simulink model "Supported_and_unsupported_combinations"  (Simulink 7.8)
settings: Solver=ode15s  StartTime=0.0  StopTime=inf  MaxStep=0.2  RelTol=1e-3
undefined symbols (not defined in the file): Engine, Engine1, Engine2, Engine3, Engine4, Engine5, Engine6, Engine7, Engine8, Engine9
libraries: sFunctionBlocks x32
(part 2 of 4)

== system Supported_and_unsupported_combinations/BoundaryConditionsConstant ==
  inflow : Inport
  Constant : Constant  Value=0
  Constant1 : Constant  Value=Pbc
  Constant2 : Constant  Value=Tbc
  Constant3 : Constant  Value=XO2bc
  Conversion_XO2_lambda : Fcn  Expr=u(1) / 0.231362 * (1 + 14.59) / (14.59 * (1 - u(1) / 0.231362))+1
  Ground : Ground
  Saturation : Saturate  UpperLimit=0.2313  LowerLimit=0
  Terminator : Terminator
  outflow : Outport
  tag scope: none=global
  wires:
  Constant1/1 -> [none]
  Constant2/1 -> [none]
  Constant3/1 -> [none], Saturation/1
  inflow/1 -> Terminator/1
  Ground/1 -> outflow/1
  Conversion_XO2_lambda/1 -> [none]
  Constant/1 -> [none]
  Saturation/1 -> Conversion_XO2_lambda/1

== system Supported_and_unsupported_combinations/BoundaryConditionsConstant1 ==
  inflow : Inport
  Constant : Constant  Value=0
  Constant1 : Constant  Value=Pbc
  Constant2 : Constant  Value=Tbc
  Constant3 : Constant  Value=XO2bc
  Conversion_XO2_lambda : Fcn  Expr=u(1) / 0.231362 * (1 + 14.59) / (14.59 * (1 - u(1) / 0.231362))+1
  Ground : Ground
  Saturation : Saturate  UpperLimit=0.2313  LowerLimit=0
  Terminator : Terminator
  outflow : Outport
  tag scope: none=global
  wires:
  Saturation/1 -> Conversion_XO2_lambda/1
  Constant/1 -> [none]
  Conversion_XO2_lambda/1 -> [none]
  Ground/1 -> outflow/1
  inflow/1 -> Terminator/1
  Constant3/1 -> Saturation/1, [none]
  Constant2/1 -> [none]
  Constant1/1 -> [none]

== system Supported_and_unsupported_combinations/BoundaryConditionsConstant2 ==
  inflow : Inport
  Constant : Constant  Value=0
  Constant1 : Constant  Value=Pbc
  Constant2 : Constant  Value=Tbc
  Constant3 : Constant  Value=XO2bc
  Conversion_XO2_lambda : Fcn  Expr=u(1) / 0.231362 * (1 + 14.59) / (14.59 * (1 - u(1) / 0.231362))+1
  Ground : Ground
  Saturation : Saturate  UpperLimit=0.2313  LowerLimit=0
  Terminator : Terminator
  outflow : Outport
  tag scope: none=global
  wires:
  Constant1/1 -> [none]
  Constant2/1 -> [none]
  Constant3/1 -> [none], Saturation/1
  inflow/1 -> Terminator/1
  Ground/1 -> outflow/1
  Conversion_XO2_lambda/1 -> [none]
  Constant/1 -> [none]
  Saturation/1 -> Conversion_XO2_lambda/1

== system Supported_and_unsupported_combinations/BoundaryConditionsConstant3 ==
  inflow : Inport
  Constant : Constant  Value=0
  Constant1 : Constant  Value=Pbc
  Constant2 : Constant  Value=Tbc
  Constant3 : Constant  Value=XO2bc
  Conversion_XO2_lambda : Fcn  Expr=u(1) / 0.231362 * (1 + 14.59) / (14.59 * (1 - u(1) / 0.231362))+1
  Ground : Ground
  Saturation : Saturate  UpperLimit=0.2313  LowerLimit=0
  Terminator : Terminator
  outflow : Outport
  tag scope: none=global
  wires:
  Saturation/1 -> Conversion_XO2_lambda/1
  Constant/1 -> [none]
  Conversion_XO2_lambda/1 -> [none]
  Ground/1 -> outflow/1
  inflow/1 -> Terminator/1
  Constant3/1 -> Saturation/1, [none]
  Constant2/1 -> [none]
  Constant1/1 -> [none]

== system Supported_and_unsupported_combinations/BoundaryConditionsConstant4 ==
  inflow : Inport
  Constant : Constant  Value=0
  Constant1 : Constant  Value=Pbc
  Constant2 : Constant  Value=Tbc
  Constant3 : Constant  Value=XO2bc
  Conversion_XO2_lambda : Fcn  Expr=u(1) / 0.231362 * (1 + 14.59) / (14.59 * (1 - u(1) / 0.231362))+1
  Ground : Ground
  Saturation : Saturate  UpperLimit=0.2313  LowerLimit=0
  Terminator : Terminator
  outflow : Outport
  tag scope: none=global
  wires:
  Constant1/1 -> [none]
  Constant2/1 -> [none]
  Constant3/1 -> [none], Saturation/1
  inflow/1 -> Terminator/1
  Ground/1 -> outflow/1
  Conversion_XO2_lambda/1 -> [none]
  Constant/1 -> [none]
  Saturation/1 -> Conversion_XO2_lambda/1

== system Supported_and_unsupported_combinations/BoundaryConditionsConstant5 ==
  inflow : Inport
  Constant : Constant  Value=0
  Constant1 : Constant  Value=Pbc
  Constant2 : Constant  Value=Tbc
  Constant3 : Constant  Value=XO2bc
  Conversion_XO2_lambda : Fcn  Expr=u(1) / 0.231362 * (1 + 14.59) / (14.59 * (1 - u(1) / 0.231362))+1
  Ground : Ground
  Saturation : Saturate  UpperLimit=0.2313  LowerLimit=0
  Terminator : Terminator
  outflow : Outport
  tag scope: none=global
  wires:
  Saturation/1 -> Conversion_XO2_lambda/1
  Constant/1 -> [none]
  Conversion_XO2_lambda/1 -> [none]
  Ground/1 -> outflow/1
  inflow/1 -> Terminator/1
  Constant3/1 -> Saturation/1, [none]
  Constant2/1 -> [none]
  Constant1/1 -> [none]

== system Supported_and_unsupported_combinations/BoundaryConditionsConstant6 ==
  inflow : Inport
  Constant : Constant  Value=0
  Constant1 : Constant  Value=Pbc
  Constant2 : Constant  Value=Tbc
  Constant3 : Constant  Value=XO2bc
  Conversion_XO2_lambda : Fcn  Expr=u(1) / 0.231362 * (1 + 14.59) / (14.59 * (1 - u(1) / 0.231362))+1
  Ground : Ground
  Saturation : Saturate  UpperLimit=0.2313  LowerLimit=0
  Terminator : Terminator
  outflow : Outport
  tag scope: none=global
  wires:
  Saturation/1 -> Conversion_XO2_lambda/1
  Constant/1 -> [none]
  Conversion_XO2_lambda/1 -> [none]
  Ground/1 -> outflow/1
  inflow/1 -> Terminator/1
  Constant3/1 -> Saturation/1, [none]
  Constant2/1 -> [none]
  Constant1/1 -> [none]

== system Supported_and_unsupported_combinations/BoundaryConditionsConstant7 ==
  inflow : Inport
  Constant : Constant  Value=0
  Constant1 : Constant  Value=Pbc
  Constant2 : Constant  Value=Tbc
  Constant3 : Constant  Value=XO2bc
  Conversion_XO2_lambda : Fcn  Expr=u(1) / 0.231362 * (1 + 14.59) / (14.59 * (1 - u(1) / 0.231362))+1
  Ground : Ground
  Saturation : Saturate  UpperLimit=0.2313  LowerLimit=0
  Terminator : Terminator
  outflow : Outport
  tag scope: none=global
  wires:
  Saturation/1 -> Conversion_XO2_lambda/1
  Constant/1 -> [none]
  Conversion_XO2_lambda/1 -> [none]
  Ground/1 -> outflow/1
  inflow/1 -> Terminator/1
  Constant3/1 -> Saturation/1, [none]
  Constant2/1 -> [none]
  Constant1/1 -> [none]

== system Supported_and_unsupported_combinations/BoundaryConditionsConstant8 ==
  inflow : Inport
  Constant : Constant  Value=0
  Constant1 : Constant  Value=Pbc
  Constant2 : Constant  Value=Tbc
  Constant3 : Constant  Value=XO2bc
  Conversion_XO2_lambda : Fcn  Expr=u(1) / 0.231362 * (1 + 14.59) / (14.59 * (1 - u(1) / 0.231362))+1
  Ground : Ground
  Saturation : Saturate  UpperLimit=0.2313  LowerLimit=0
  Terminator : Terminator
  outflow : Outport
  tag scope: none=global
  wires:
  Constant1/1 -> [none]
  Constant2/1 -> [none]
  Constant3/1 -> [none], Saturation/1
  inflow/1 -> Terminator/1
  Ground/1 -> outflow/1
  Conversion_XO2_lambda/1 -> [none]
  Constant/1 -> [none]
  Saturation/1 -> Conversion_XO2_lambda/1

== system Supported_and_unsupported_combinations/BoundaryConditionsConstant9 ==
  inflow : Inport
  Constant : Constant  Value=0
  Constant1 : Constant  Value=Pbc
  Constant2 : Constant  Value=Tbc
  Constant3 : Constant  Value=XO2bc
  Conversion_XO2_lambda : Fcn  Expr=u(1) / 0.231362 * (1 + 14.59) / (14.59 * (1 - u(1) / 0.231362))+1
  Ground : Ground
  Saturation : Saturate  UpperLimit=0.2313  LowerLimit=0
  Terminator : Terminator
  outflow : Outport
  tag scope: none=global
  wires:
  Constant1/1 -> [none]
  Constant2/1 -> [none]
  Constant3/1 -> [none], Saturation/1
  inflow/1 -> Terminator/1
  Ground/1 -> outflow/1
  Conversion_XO2_lambda/1 -> [none]
  Constant/1 -> [none]
  Saturation/1 -> Conversion_XO2_lambda/1

== system Supported_and_unsupported_combinations/Engine ==
  inflow : Inport
  OmegaEng : Inport  Port=2
  IQ : Inport  Port=3
  uSOI : Inport  Port=4
  uPR : Inport  Port=5
  Constant : Constant  Value=0
  Constant1 : Constant  Value=0
  Engine : Subsystem
  ExhaustManifold : Subsystem
  IntakeManifold : Subsystem
  outflow : Outport
  tag scope: Engine_EngineSpeed=global, Engine_FuelMassflow=global
  wires:
  uPR/1 -> Engine/10(uPR)
  Constant/1 -> Engine/9(uECA)
  Constant1/1 -> Engine/8(uICA)
  Engine/5(Mfuel) -> ExhaustManifold/5(Mfuel), [Engine_FuelMassflow]
  Engine/4(outflow) -> ExhaustManifold/4(inflow)
  IntakeManifold/3(outflow) -> Engine/4(inflow)
  IntakeManifold/1(Pim) -> Engine/1(Pin)
  ExhaustManifold/1(Pout) -> Engine/2(Pout)
  Engine/3(XO2out) -> ExhaustManifold/3(XO2in)
  IntakeManifold/2(XO2out) -> Engine/3(XO2in)
  Engine/2(Tout) -> ExhaustManifold/2(Tin)
  Engine/1(Meng) -> IntakeManifold/1(Mout), ExhaustManifold/1(Meng)
  ExhaustManifold/2(outflow) -> outflow/1
  inflow/1 -> IntakeManifold/2(inflow)
  OmegaEng/1 -> Engine/5(OmegaEng), [Engine_EngineSpeed]
  uSOI/1 -> Engine/7(uSOI)
  IQ/1 -> Engine/6(IQ)

== system Supported_and_unsupported_combinations/Engine1 ==
  inflow : Inport
  OmegaEng : Inport  Port=2
  IQ : Inport  Port=3
  uSOI : Inport  Port=4
  uPR : Inport  Port=5
  Constant : Constant  Value=0
  Constant1 : Constant  Value=0
  Engine : Subsystem
  ExhaustManifold : Subsystem
  IntakeManifold : Subsystem
  outflow : Outport
  tag scope: Engine_EngineSpeed=global, Engine_FuelMassflow=global
  wires:
  IQ/1 -> Engine/6(IQ)
  uSOI/1 -> Engine/7(uSOI)
  OmegaEng/1 -> [Engine_EngineSpeed], Engine/5(OmegaEng)
  inflow/1 -> IntakeManifold/2(inflow)
  ExhaustManifold/2(outflow) -> outflow/1
  Engine/1(Meng) -> ExhaustManifold/1(Meng), IntakeManifold/1(Mout)
  Engine/2(Tout) -> ExhaustManifold/2(Tin)
  IntakeManifold/2(XO2out) -> Engine/3(XO2in)
  Engine/3(XO2out) -> ExhaustManifold/3(XO2in)
  ExhaustManifold/1(Pout) -> Engine/2(Pout)
  IntakeManifold/1(Pim) -> Engine/1(Pin)
  IntakeManifold/3(outflow) -> Engine/4(inflow)
  Engine/4(outflow) -> ExhaustManifold/4(inflow)
  Engine/5(Mfuel) -> [Engine_FuelMassflow], ExhaustManifold/5(Mfuel)
  Constant1/1 -> Engine/8(uICA)
  Constant/1 -> Engine/9(uECA)
  uPR/1 -> Engine/10(uPR)

== system Supported_and_unsupported_combinations/Engine2 ==
  inflow : Inport
  OmegaEng : Inport  Port=2
  IQ : Inport  Port=3
  uSOI : Inport  Port=4
  uPR : Inport  Port=5
  Constant : Constant  Value=0
  Constant1 : Constant  Value=0
  Engine : Subsystem
  ExhaustManifold : Subsystem
  IntakeManifold : Subsystem
  outflow : Outport
  tag scope: Engine_EngineSpeed=global, Engine_FuelMassflow=global
  wires:
  IQ/1 -> Engine/6(IQ)
  uSOI/1 -> Engine/7(uSOI)
  OmegaEng/1 -> [Engine_EngineSpeed], Engine/5(OmegaEng)
  inflow/1 -> IntakeManifold/2(inflow)
  ExhaustManifold/2(outflow) -> outflow/1
  Engine/1(Meng) -> ExhaustManifold/1(Meng), IntakeManifold/1(Mout)
  Engine/2(Tout) -> ExhaustManifold/2(Tin)
  IntakeManifold/2(XO2out) -> Engine/3(XO2in)
  Engine/3(XO2out) -> ExhaustManifold/3(XO2in)
  ExhaustManifold/1(Pout) -> Engine/2(Pout)
  IntakeManifold/1(Pim) -> Engine/1(Pin)
  IntakeManifold/3(outflow) -> Engine/4(inflow)
  Engine/4(outflow) -> ExhaustManifold/4(inflow)
  Engine/5(Mfuel) -> [Engine_FuelMassflow], ExhaustManifold/5(Mfuel)
  Constant1/1 -> Engine/8(uICA)
  Constant/1 -> Engine/9(uECA)
  uPR/1 -> Engine/10(uPR)

== system Supported_and_unsupported_combinations/Engine3 ==
  inflow : Inport
  OmegaEng : Inport  Port=2
  IQ : Inport  Port=3
  uSOI : Inport  Port=4
  uPR : Inport  Port=5
  Constant : Constant  Value=0
  Constant1 : Constant  Value=0
  Engine : Subsystem
  ExhaustManifold : Subsystem
  IntakeManifold : Subsystem
  outflow : Outport
  tag scope: Engine_EngineSpeed=global, Engine_FuelMassflow=global
  wires:
  uPR/1 -> Engine/10(uPR)
  Constant/1 -> Engine/9(uECA)
  Constant1/1 -> Engine/8(uICA)
  Engine/5(Mfuel) -> ExhaustManifold/5(Mfuel), [Engine_FuelMassflow]
  Engine/4(outflow) -> ExhaustManifold/4(inflow)
  IntakeManifold/3(outflow) -> Engine/4(inflow)
  IntakeManifold/1(Pim) -> Engine/1(Pin)
  ExhaustManifold/1(Pout) -> Engine/2(Pout)
  Engine/3(XO2out) -> ExhaustManifold/3(XO2in)
  IntakeManifold/2(XO2out) -> Engine/3(XO2in)
  Engine/2(Tout) -> ExhaustManifold/2(Tin)
  Engine/1(Meng) -> IntakeManifold/1(Mout), ExhaustManifold/1(Meng)
  ExhaustManifold/2(outflow) -> outflow/1
  inflow/1 -> IntakeManifold/2(inflow)
  OmegaEng/1 -> Engine/5(OmegaEng), [Engine_EngineSpeed]
  uSOI/1 -> Engine/7(uSOI)
  IQ/1 -> Engine/6(IQ)

== system Supported_and_unsupported_combinations/Engine4 ==
  inflow : Inport
  OmegaEng : Inport  Port=2
  IQ : Inport  Port=3
  uSOI : Inport  Port=4
  uPR : Inport  Port=5
  Constant : Constant  Value=0
  Constant1 : Constant  Value=0
  Engine : Subsystem
  ExhaustManifold : Subsystem
  IntakeManifold : Subsystem
  outflow : Outport
  tag scope: Engine_EngineSpeed=global, Engine_FuelMassflow=global
  wires:
  IQ/1 -> Engine/6(IQ)
  uSOI/1 -> Engine/7(uSOI)
  OmegaEng/1 -> [Engine_EngineSpeed], Engine/5(OmegaEng)
  inflow/1 -> IntakeManifold/2(inflow)
  ExhaustManifold/2(outflow) -> outflow/1
  Engine/1(Meng) -> ExhaustManifold/1(Meng), IntakeManifold/1(Mout)
  Engine/2(Tout) -> ExhaustManifold/2(Tin)
  IntakeManifold/2(XO2out) -> Engine/3(XO2in)
  Engine/3(XO2out) -> ExhaustManifold/3(XO2in)
  ExhaustManifold/1(Pout) -> Engine/2(Pout)
  IntakeManifold/1(Pim) -> Engine/1(Pin)
  IntakeManifold/3(outflow) -> Engine/4(inflow)
  Engine/4(outflow) -> ExhaustManifold/4(inflow)
  Engine/5(Mfuel) -> [Engine_FuelMassflow], ExhaustManifold/5(Mfuel)
  Constant1/1 -> Engine/8(uICA)
  Constant/1 -> Engine/9(uECA)
  uPR/1 -> Engine/10(uPR)

== system Supported_and_unsupported_combinations/Engine5 ==
  inflow : Inport
  OmegaEng : Inport  Port=2
  IQ : Inport  Port=3
  uSOI : Inport  Port=4
  uPR : Inport  Port=5
  Constant : Constant  Value=0
  Constant1 : Constant  Value=0
  Engine : Subsystem
  ExhaustManifold : Subsystem
  IntakeManifold : Subsystem
  outflow : Outport
  tag scope: Engine_EngineSpeed=global, Engine_FuelMassflow=global
  wires:
  uPR/1 -> Engine/10(uPR)
  Constant/1 -> Engine/9(uECA)
  Constant1/1 -> Engine/8(uICA)
  Engine/5(Mfuel) -> ExhaustManifold/5(Mfuel), [Engine_FuelMassflow]
  Engine/4(outflow) -> ExhaustManifold/4(inflow)
  IntakeManifold/3(outflow) -> Engine/4(inflow)
  IntakeManifold/1(Pim) -> Engine/1(Pin)
  ExhaustManifold/1(Pout) -> Engine/2(Pout)
  Engine/3(XO2out) -> ExhaustManifold/3(XO2in)
  IntakeManifold/2(XO2out) -> Engine/3(XO2in)
  Engine/2(Tout) -> ExhaustManifold/2(Tin)
  Engine/1(Meng) -> IntakeManifold/1(Mout), ExhaustManifold/1(Meng)
  ExhaustManifold/2(outflow) -> outflow/1
  inflow/1 -> IntakeManifold/2(inflow)
  OmegaEng/1 -> Engine/5(OmegaEng), [Engine_EngineSpeed]
  uSOI/1 -> Engine/7(uSOI)
  IQ/1 -> Engine/6(IQ)

== system Supported_and_unsupported_combinations/Engine6 ==
  inflow : Inport
  OmegaEng : Inport  Port=2
  IQ : Inport  Port=3
  uSOI : Inport  Port=4
  uPR : Inport  Port=5
  Constant : Constant  Value=0
  Constant1 : Constant  Value=0
  Engine : Subsystem
  ExhaustManifold : Subsystem
  IntakeManifold : Subsystem
  outflow : Outport
  tag scope: Engine_EngineSpeed=global, Engine_FuelMassflow=global
  wires:
  uPR/1 -> Engine/10(uPR)
  Constant/1 -> Engine/9(uECA)
  Constant1/1 -> Engine/8(uICA)
  Engine/5(Mfuel) -> ExhaustManifold/5(Mfuel), [Engine_FuelMassflow]
  Engine/4(outflow) -> ExhaustManifold/4(inflow)
  IntakeManifold/3(outflow) -> Engine/4(inflow)
  IntakeManifold/1(Pim) -> Engine/1(Pin)
  ExhaustManifold/1(Pout) -> Engine/2(Pout)
  Engine/3(XO2out) -> ExhaustManifold/3(XO2in)
  IntakeManifold/2(XO2out) -> Engine/3(XO2in)
  Engine/2(Tout) -> ExhaustManifold/2(Tin)
  Engine/1(Meng) -> IntakeManifold/1(Mout), ExhaustManifold/1(Meng)
  ExhaustManifold/2(outflow) -> outflow/1
  inflow/1 -> IntakeManifold/2(inflow)
  OmegaEng/1 -> Engine/5(OmegaEng), [Engine_EngineSpeed]
  uSOI/1 -> Engine/7(uSOI)
  IQ/1 -> Engine/6(IQ)

== system Supported_and_unsupported_combinations/Engine7 ==
  inflow : Inport
  OmegaEng : Inport  Port=2
  IQ : Inport  Port=3
  uSOI : Inport  Port=4
  uPR : Inport  Port=5
  Constant : Constant  Value=0
  Constant1 : Constant  Value=0
  Engine : Subsystem
  ExhaustManifold : Subsystem
  IntakeManifold : Subsystem
  outflow : Outport
  tag scope: Engine_EngineSpeed=global, Engine_FuelMassflow=global
  wires:
  IQ/1 -> Engine/6(IQ)
  uSOI/1 -> Engine/7(uSOI)
  OmegaEng/1 -> [Engine_EngineSpeed], Engine/5(OmegaEng)
  inflow/1 -> IntakeManifold/2(inflow)
  ExhaustManifold/2(outflow) -> outflow/1
  Engine/1(Meng) -> ExhaustManifold/1(Meng), IntakeManifold/1(Mout)
  Engine/2(Tout) -> ExhaustManifold/2(Tin)
  IntakeManifold/2(XO2out) -> Engine/3(XO2in)
  Engine/3(XO2out) -> ExhaustManifold/3(XO2in)
  ExhaustManifold/1(Pout) -> Engine/2(Pout)
  IntakeManifold/1(Pim) -> Engine/1(Pin)
  IntakeManifold/3(outflow) -> Engine/4(inflow)
  Engine/4(outflow) -> ExhaustManifold/4(inflow)
  Engine/5(Mfuel) -> [Engine_FuelMassflow], ExhaustManifold/5(Mfuel)
  Constant1/1 -> Engine/8(uICA)
  Constant/1 -> Engine/9(uECA)
  uPR/1 -> Engine/10(uPR)

== system Supported_and_unsupported_combinations/Engine8 ==
  inflow : Inport
  OmegaEng : Inport  Port=2
  IQ : Inport  Port=3
  uSOI : Inport  Port=4
  uPR : Inport  Port=5
  Constant : Constant  Value=0
  Constant1 : Constant  Value=0
  Engine : Subsystem
  ExhaustManifold : Subsystem
  IntakeManifold : Subsystem
  outflow : Outport
  tag scope: Engine_EngineSpeed=global, Engine_FuelMassflow=global
  wires:
  uPR/1 -> Engine/10(uPR)
  Constant/1 -> Engine/9(uECA)
  Constant1/1 -> Engine/8(uICA)
  Engine/5(Mfuel) -> ExhaustManifold/5(Mfuel), [Engine_FuelMassflow]
  Engine/4(outflow) -> ExhaustManifold/4(inflow)
  IntakeManifold/3(outflow) -> Engine/4(inflow)
  IntakeManifold/1(Pim) -> Engine/1(Pin)
  ExhaustManifold/1(Pout) -> Engine/2(Pout)
  Engine/3(XO2out) -> ExhaustManifold/3(XO2in)
  IntakeManifold/2(XO2out) -> Engine/3(XO2in)
  Engine/2(Tout) -> ExhaustManifold/2(Tin)
  Engine/1(Meng) -> IntakeManifold/1(Mout), ExhaustManifold/1(Meng)
  ExhaustManifold/2(outflow) -> outflow/1
  inflow/1 -> IntakeManifold/2(inflow)
  OmegaEng/1 -> Engine/5(OmegaEng), [Engine_EngineSpeed]
  uSOI/1 -> Engine/7(uSOI)
  IQ/1 -> Engine/6(IQ)

== system Supported_and_unsupported_combinations/Engine9 ==
  inflow : Inport
  OmegaEng : Inport  Port=2
  IQ : Inport  Port=3
  uSOI : Inport  Port=4
  uPR : Inport  Port=5
  Constant : Constant  Value=0
  Constant1 : Constant  Value=0
  Engine : Subsystem
  ExhaustManifold : Subsystem
  IntakeManifold : Subsystem
  outflow : Outport
  tag scope: Engine_EngineSpeed=global, Engine_FuelMassflow=global
  wires:
  IQ/1 -> Engine/6(IQ)
  uSOI/1 -> Engine/7(uSOI)
  OmegaEng/1 -> [Engine_EngineSpeed], Engine/5(OmegaEng)
  inflow/1 -> IntakeManifold/2(inflow)
  ExhaustManifold/2(outflow) -> outflow/1
  Engine/1(Meng) -> ExhaustManifold/1(Meng), IntakeManifold/1(Mout)
  Engine/2(Tout) -> ExhaustManifold/2(Tin)
  IntakeManifold/2(XO2out) -> Engine/3(XO2in)
  Engine/3(XO2out) -> ExhaustManifold/3(XO2in)
  ExhaustManifold/1(Pout) -> Engine/2(Pout)
  IntakeManifold/1(Pim) -> Engine/1(Pin)
  IntakeManifold/3(outflow) -> Engine/4(inflow)
  Engine/4(outflow) -> ExhaustManifold/4(inflow)
  Engine/5(Mfuel) -> [Engine_FuelMassflow], ExhaustManifold/5(Mfuel)
  Constant1/1 -> Engine/8(uICA)
  Constant/1 -> Engine/9(uECA)
  uPR/1 -> Engine/10(uPR)

== system Supported_and_unsupported_combinations/FlowRestriction ==
  inflow : Inport
  AuxiliaryManifold : sFunctionBlocks/AuxiliaryManifold  Tag=isAuxManifold  V=1  R=288  Cp=1020  pinit=1e5  isActive=0
  Constant : Constant
  FlowRestriction : sFunctionBlocks/FlowRestriction  ParRestr=[4.77193819761005 2.93887546670532]  R=288
  Product1 : Product  RndMeth=Zero
  Switch : Switch  Criteria=u2 > Threshold
  outflow : Outport
  tag scope: none=global
  wires:
  [none] -> Product1/2
  Product1/1 -> [none]
  Constant/1 -> Switch/2
  [none] -> FlowRestriction/2
  Switch/1 -> FlowRestriction/1
  AuxiliaryManifold/1 -> Switch/1, [none]
  [none] -> FlowRestriction/3, AuxiliaryManifold/3
  FlowRestriction/1 -> AuxiliaryManifold/2, Product1/1, [none]
  inflow/1 -> outflow/1  "flow"
  [none] -> AuxiliaryManifold/1
  [none] -> Switch/3

== system Supported_and_unsupported_combinations/FlowRestriction1 ==
  inflow : Inport
  AuxiliaryManifold : sFunctionBlocks/AuxiliaryManifold  Tag=isAuxManifold  V=1  R=288  Cp=1020  pinit=1e5  isActive=0
  Constant : Constant
  FlowRestriction : sFunctionBlocks/FlowRestriction  ParRestr=[4.77193819761005 2.93887546670532]  R=288
  Product1 : Product  RndMeth=Zero
  Switch : Switch  Criteria=u2 > Threshold
  outflow : Outport
  tag scope: none=global
  wires:
  [none] -> Switch/3
  [none] -> AuxiliaryManifold/1
  inflow/1 -> outflow/1  "flow"
  FlowRestriction/1 -> [none], Product1/1, AuxiliaryManifold/2
  [none] -> AuxiliaryManifold/3, FlowRestriction/3
  AuxiliaryManifold/1 -> [none], Switch/1
  Switch/1 -> FlowRestriction/1
  [none] -> FlowRestriction/2
  Constant/1 -> Switch/2
  Product1/1 -> [none]
  [none] -> Product1/2

== system Supported_and_unsupported_combinations/FlowRestriction2 ==
  inflow : Inport
  AuxiliaryManifold : sFunctionBlocks/AuxiliaryManifold  Tag=isAuxManifold  V=1  R=288  Cp=1020  pinit=1e5  isActive=0
  Constant : Constant
  FlowRestriction : sFunctionBlocks/FlowRestriction  ParRestr=[4.77193819761005 2.93887546670532]  R=288
  Product1 : Product  RndMeth=Zero
  Switch : Switch  Criteria=u2 > Threshold
  outflow : Outport
  tag scope: none=global
  wires:
  [none] -> Product1/2
  Product1/1 -> [none]
  Constant/1 -> Switch/2
  [none] -> FlowRestriction/2
  Switch/1 -> FlowRestriction/1
  AuxiliaryManifold/1 -> Switch/1, [none]
  [none] -> FlowRestriction/3, AuxiliaryManifold/3
  FlowRestriction/1 -> AuxiliaryManifold/2, Product1/1, [none]
  inflow/1 -> outflow/1  "flow"
  [none] -> AuxiliaryManifold/1
  [none] -> Switch/3

== system Supported_and_unsupported_combinations/FlowRestriction3 ==
  inflow : Inport
  AuxiliaryManifold : sFunctionBlocks/AuxiliaryManifold  Tag=isAuxManifold  V=1  R=288  Cp=1020  pinit=1e5  isActive=0
  Constant : Constant
  FlowRestriction : sFunctionBlocks/FlowRestriction  ParRestr=[4.77193819761005 2.93887546670532]  R=288
  Product1 : Product  RndMeth=Zero
  Switch : Switch  Criteria=u2 > Threshold
  outflow : Outport
  tag scope: none=global
  wires:
  [none] -> Switch/3
  [none] -> AuxiliaryManifold/1
  inflow/1 -> outflow/1  "flow"
  FlowRestriction/1 -> [none], Product1/1, AuxiliaryManifold/2
  [none] -> AuxiliaryManifold/3, FlowRestriction/3
  AuxiliaryManifold/1 -> [none], Switch/1
  Switch/1 -> FlowRestriction/1
  [none] -> FlowRestriction/2
  Constant/1 -> Switch/2
  Product1/1 -> [none]
  [none] -> Product1/2

== system Supported_and_unsupported_combinations/FlowRestriction4 ==
  inflow : Inport
  AuxiliaryManifold : sFunctionBlocks/AuxiliaryManifold  Tag=isAuxManifold  V=1  R=288  Cp=1020  pinit=1e5  isActive=0
  Constant : Constant
  FlowRestriction : sFunctionBlocks/FlowRestriction  ParRestr=[4.77193819761005 2.93887546670532]  R=288
  Product1 : Product  RndMeth=Zero
  Switch : Switch  Criteria=u2 > Threshold
  outflow : Outport
  tag scope: none=global
  wires:
  [none] -> Product1/2
  Product1/1 -> [none]
  Constant/1 -> Switch/2
  [none] -> FlowRestriction/2
  Switch/1 -> FlowRestriction/1
  AuxiliaryManifold/1 -> Switch/1, [none]
  [none] -> FlowRestriction/3, AuxiliaryManifold/3
  FlowRestriction/1 -> AuxiliaryManifold/2, Product1/1, [none]
  inflow/1 -> outflow/1  "flow"
  [none] -> AuxiliaryManifold/1
  [none] -> Switch/3

== system Supported_and_unsupported_combinations/FlowRestriction5 ==
  inflow : Inport
  AuxiliaryManifold : sFunctionBlocks/AuxiliaryManifold  Tag=isAuxManifold  V=1  R=288  Cp=1020  pinit=1e5  isActive=0
  Constant : Constant
  FlowRestriction : sFunctionBlocks/FlowRestriction  ParRestr=[4.77193819761005 2.93887546670532]  R=288
  Product1 : Product  RndMeth=Zero
  Switch : Switch  Criteria=u2 > Threshold
  outflow : Outport
  tag scope: none=global
  wires:
  [none] -> Switch/3
  [none] -> AuxiliaryManifold/1
  inflow/1 -> outflow/1  "flow"
  FlowRestriction/1 -> [none], Product1/1, AuxiliaryManifold/2
  [none] -> AuxiliaryManifold/3, FlowRestriction/3
  AuxiliaryManifold/1 -> [none], Switch/1
  Switch/1 -> FlowRestriction/1
  [none] -> FlowRestriction/2
  Constant/1 -> Switch/2
  Product1/1 -> [none]
  [none] -> Product1/2

== system Supported_and_unsupported_combinations/FlowRestriction6 ==
  inflow : Inport
  AuxiliaryManifold : sFunctionBlocks/AuxiliaryManifold  Tag=isAuxManifold  V=1  R=288  Cp=1020  pinit=1e5  isActive=0
  Constant : Constant
  FlowRestriction : sFunctionBlocks/FlowRestriction  ParRestr=[4.77193819761005 2.93887546670532]  R=288
  Product1 : Product  RndMeth=Zero
  Switch : Switch  Criteria=u2 > Threshold
  outflow : Outport
  tag scope: none=global
  wires:
  [none] -> Product1/2
  Product1/1 -> [none]
  Constant/1 -> Switch/2
  [none] -> FlowRestriction/2
  Switch/1 -> FlowRestriction/1
  AuxiliaryManifold/1 -> Switch/1, [none]
  [none] -> FlowRestriction/3, AuxiliaryManifold/3
  FlowRestriction/1 -> AuxiliaryManifold/2, Product1/1, [none]
  inflow/1 -> outflow/1  "flow"
  [none] -> AuxiliaryManifold/1
  [none] -> Switch/3

== system Supported_and_unsupported_combinations/FlowRestriction7 ==
  inflow : Inport
  AuxiliaryManifold : sFunctionBlocks/AuxiliaryManifold  Tag=isAuxManifold  V=1  R=288  Cp=1020  pinit=1e5  isActive=0
  Constant : Constant
  FlowRestriction : sFunctionBlocks/FlowRestriction  ParRestr=[4.77193819761005 2.93887546670532]  R=288
  Product1 : Product  RndMeth=Zero
  Switch : Switch  Criteria=u2 > Threshold
  outflow : Outport
  tag scope: none=global
  wires:
  [none] -> Switch/3
  [none] -> AuxiliaryManifold/1
  inflow/1 -> outflow/1  "flow"
  FlowRestriction/1 -> [none], Product1/1, AuxiliaryManifold/2
  [none] -> AuxiliaryManifold/3, FlowRestriction/3
  AuxiliaryManifold/1 -> [none], Switch/1
  Switch/1 -> FlowRestriction/1
  [none] -> FlowRestriction/2
  Constant/1 -> Switch/2
  Product1/1 -> [none]
  [none] -> Product1/2

== system Supported_and_unsupported_combinations/FlowSplitter ==
  inflow : Inport
  OutFlow1 : Subsystem  Tag=isFlowSplitter
  OutFlow2 : Subsystem  Tag=isFlowSplitter
  TotalOutFlow : Subsystem
  outflow1 : Outport
  outflow2 : Outport  Port=2
  wires:
  inflow/1 -> TotalOutFlow/3(inflow)
  OutFlow1/2(outflow) -> outflow1/1
  TotalOutFlow/1(outflow) -> OutFlow1/1(inflow), OutFlow2/1(inflow)
  OutFlow1/1(Mout1) -> TotalOutFlow/1(Mout1)
  OutFlow2/2(outflow) -> outflow2/1
  OutFlow2/1(Mout2) -> TotalOutFlow/2(Mout2)

== system Supported_and_unsupported_combinations/FlowSplitter1 ==
  inflow : Inport
  OutFlow1 : Subsystem  Tag=isFlowSplitter
  OutFlow2 : Subsystem  Tag=isFlowSplitter
  TotalOutFlow : Subsystem
  outflow1 : Outport
  outflow2 : Outport  Port=2
  wires:
  OutFlow2/1(Mout2) -> TotalOutFlow/2(Mout2)
  OutFlow2/2(outflow) -> outflow2/1
  OutFlow1/1(Mout1) -> TotalOutFlow/1(Mout1)
  TotalOutFlow/1(outflow) -> OutFlow2/1(inflow), OutFlow1/1(inflow)
  OutFlow1/2(outflow) -> outflow1/1
  inflow/1 -> TotalOutFlow/3(inflow)

== system Supported_and_unsupported_combinations/FlowSplitter2 ==
  inflow : Inport
  OutFlow1 : Subsystem  Tag=isFlowSplitter
  OutFlow2 : Subsystem  Tag=isFlowSplitter
  TotalOutFlow : Subsystem
  outflow1 : Outport
  outflow2 : Outport  Port=2
  wires:
  OutFlow2/1(Mout2) -> TotalOutFlow/2(Mout2)
  OutFlow2/2(outflow) -> outflow2/1
  OutFlow1/1(Mout1) -> TotalOutFlow/1(Mout1)
  TotalOutFlow/1(outflow) -> OutFlow2/1(inflow), OutFlow1/1(inflow)
  OutFlow1/2(outflow) -> outflow1/1
  inflow/1 -> TotalOutFlow/3(inflow)

== system Supported_and_unsupported_combinations/FlowSplitter3 ==
  inflow : Inport
  OutFlow1 : Subsystem  Tag=isFlowSplitter
  OutFlow2 : Subsystem  Tag=isFlowSplitter
  TotalOutFlow : Subsystem
  outflow1 : Outport
  outflow2 : Outport  Port=2
  wires:
  inflow/1 -> TotalOutFlow/3(inflow)
  OutFlow1/2(outflow) -> outflow1/1
  TotalOutFlow/1(outflow) -> OutFlow1/1(inflow), OutFlow2/1(inflow)
  OutFlow1/1(Mout1) -> TotalOutFlow/1(Mout1)
  OutFlow2/2(outflow) -> outflow2/1
  OutFlow2/1(Mout2) -> TotalOutFlow/2(Mout2)

== system Supported_and_unsupported_combinations/HeatExchanger ==
  inflow : Inport
  HeatExchanger : sFunctionBlocks/HeatExchanger  Tsink=314.918321500236  ParCoolingEff=0.521897247893149
  LoopCutter : TransferFcn  Denominator=[0.00001 1]
  outflow : Outport
  tag scope: none=global
  wires:
  [none] -> LoopCutter/1
  LoopCutter/1 -> HeatExchanger/2
  HeatExchanger/1 -> [none]
  [none] -> HeatExchanger/1
  inflow/1 -> outflow/1  "flow"

== system Supported_and_unsupported_combinations/HeatExchanger1 ==
  inflow : Inport
  HeatExchanger : sFunctionBlocks/HeatExchanger  Tsink=314.918321500236  ParCoolingEff=0.521897247893149
  LoopCutter : TransferFcn  Denominator=[0.00001 1]
  outflow : Outport
  tag scope: none=global
  wires:
  inflow/1 -> outflow/1  "flow"
  [none] -> HeatExchanger/1
  HeatExchanger/1 -> [none]
  LoopCutter/1 -> HeatExchanger/2
  [none] -> LoopCutter/1

== system Supported_and_unsupported_combinations/HeatExchanger2 ==
  inflow : Inport
  HeatExchanger : sFunctionBlocks/HeatExchanger  Tsink=314.918321500236  ParCoolingEff=0.521897247893149
  LoopCutter : TransferFcn  Denominator=[0.00001 1]
  outflow : Outport
  tag scope: none=global
  wires:
  inflow/1 -> outflow/1  "flow"
  [none] -> HeatExchanger/1
  HeatExchanger/1 -> [none]
  LoopCutter/1 -> HeatExchanger/2
  [none] -> LoopCutter/1

== system Supported_and_unsupported_combinations/HeatExchanger3 ==
  inflow : Inport
  HeatExchanger : sFunctionBlocks/HeatExchanger  Tsink=314.918321500236  ParCoolingEff=0.521897247893149
  LoopCutter : TransferFcn  Denominator=[0.00001 1]
  outflow : Outport
  tag scope: none=global
  wires:
  [none] -> LoopCutter/1
  LoopCutter/1 -> HeatExchanger/2
  HeatExchanger/1 -> [none]
  [none] -> HeatExchanger/1
  inflow/1 -> outflow/1  "flow"

== system Supported_and_unsupported_combinations/Mix ==
  inflow1 : Inport
  inflow2 : Inport  Port=2
  InFlow1 : Subsystem
  InFlow2 : Subsystem
  TotalInFlow : Subsystem  Tag=isMixing
  outflow : Outport
  wires:
  TotalInFlow/1(outflow) -> outflow/1
  InFlow2/2(Min) -> TotalInFlow/4(Min2)
  InFlow1/2(Min) -> TotalInFlow/1(Min1)
  InFlow2/4(outflow) -> TotalInFlow/8(inflow2)
  InFlow1/4(outflow) -> TotalInFlow/7(inflow1)
  inflow2/1 -> InFlow2/1(inflow)
  inflow1/1 -> InFlow1/1(inflow)
  InFlow2/3(XO2in) -> TotalInFlow/6(XO2in2)
  InFlow1/3(XO2in) -> TotalInFlow/5(XO2in1)
  InFlow2/1(Tin) -> TotalInFlow/3(Tin2)
  InFlow1/1(Tin) -> TotalInFlow/2(Tin1)

== system Supported_and_unsupported_combinations/Mix1 ==
  inflow1 : Inport
  inflow2 : Inport  Port=2
  InFlow1 : Subsystem
  InFlow2 : Subsystem
  TotalInFlow : Subsystem  Tag=isMixing
  outflow : Outport
  wires:
  InFlow1/1(Tin) -> TotalInFlow/2(Tin1)
  InFlow2/1(Tin) -> TotalInFlow/3(Tin2)
  InFlow1/3(XO2in) -> TotalInFlow/5(XO2in1)
  InFlow2/3(XO2in) -> TotalInFlow/6(XO2in2)
  inflow1/1 -> InFlow1/1(inflow)
  inflow2/1 -> InFlow2/1(inflow)
  InFlow1/4(outflow) -> TotalInFlow/7(inflow1)
  InFlow2/4(outflow) -> TotalInFlow/8(inflow2)
  InFlow1/2(Min) -> TotalInFlow/1(Min1)
  InFlow2/2(Min) -> TotalInFlow/4(Min2)
  TotalInFlow/1(outflow) -> outflow/1

== system Supported_and_unsupported_combinations/Mix2 ==
  inflow1 : Inport
  inflow2 : Inport  Port=2
  InFlow1 : Subsystem
  InFlow2 : Subsystem
  TotalInFlow : Subsystem  Tag=isMixing
  outflow : Outport
  wires:
  InFlow1/1(Tin) -> TotalInFlow/2(Tin1)
  InFlow2/1(Tin) -> TotalInFlow/3(Tin2)
  InFlow1/3(XO2in) -> TotalInFlow/5(XO2in1)
  InFlow2/3(XO2in) -> TotalInFlow/6(XO2in2)
  inflow1/1 -> InFlow1/1(inflow)
  inflow2/1 -> InFlow2/1(inflow)
  InFlow1/4(outflow) -> TotalInFlow/7(inflow1)
  InFlow2/4(outflow) -> TotalInFlow/8(inflow2)
  InFlow1/2(Min) -> TotalInFlow/1(Min1)
  InFlow2/2(Min) -> TotalInFlow/4(Min2)
  TotalInFlow/1(outflow) -> outflow/1

== system Supported_and_unsupported_combinations/Mix3 ==
  inflow1 : Inport
  inflow2 : Inport  Port=2
  InFlow1 : Subsystem
  InFlow2 : Subsystem
  TotalInFlow : Subsystem  Tag=isMixing
  outflow : Outport
  wires:
  TotalInFlow/1(outflow) -> outflow/1
  InFlow2/2(Min) -> TotalInFlow/4(Min2)
  InFlow1/2(Min) -> TotalInFlow/1(Min1)
  InFlow2/4(outflow) -> TotalInFlow/8(inflow2)
  InFlow1/4(outflow) -> TotalInFlow/7(inflow1)
  inflow2/1 -> InFlow2/1(inflow)
  inflow1/1 -> InFlow1/1(inflow)
  InFlow2/3(XO2in) -> TotalInFlow/6(XO2in2)
  InFlow1/3(XO2in) -> TotalInFlow/5(XO2in1)
  InFlow2/1(Tin) -> TotalInFlow/3(Tin2)
  InFlow1/1(Tin) -> TotalInFlow/2(Tin1)

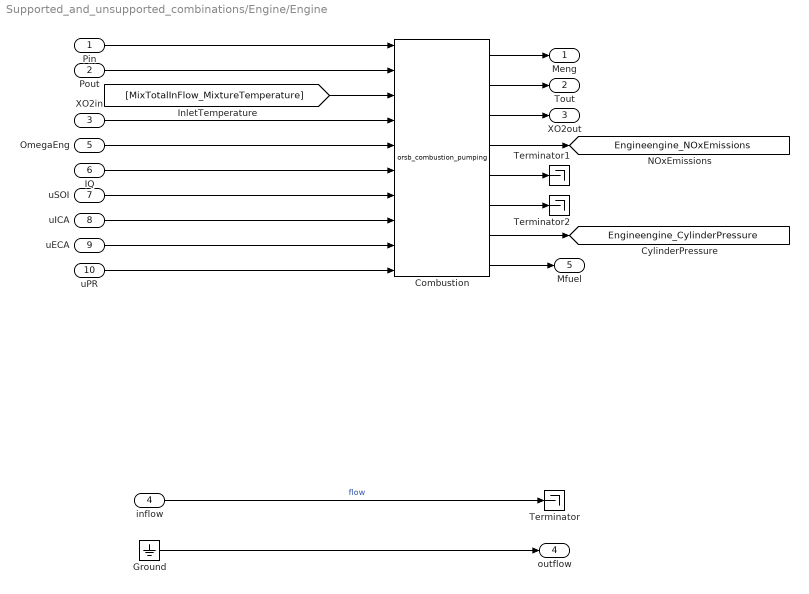
== system Supported_and_unsupported_combinations/Engine/Engine ==
  Pin : Inport
  Pout : Inport  Port=2
  XO2in : Inport  Port=3
  inflow : Inport  Port=4
  OmegaEng : Inport  Port=5
  IQ : Inport  Port=6
  uSOI : Inport  Port=7
  uICA : Inport  Port=8
  uECA : Inport  Port=9
  uPR : Inport  Port=10
  Combustion : S-Function  FunctionName=orsb_combustion_pumping  Parameters=Displ, CompRatio, Ncyl, ValveMdl, TmpMdl, IgnitMdl, PressMdl, Cp, Cv, port_num_NOx, NOxMdl,  EnableBusSupport=off  mask(combustion_pumping){Displ=12.9, CompRatio=18, Ncyl=6, ValveMdl=[0.00961171539106083 -0.172384589641163], TmpMdl=[-0.025503095647334 0.175522235872159 0.0255043476751577 0.0373865335774022 0], IgnitMdl=[0.484351292851209 0.143524113288744 -0.055676015193126 -0.0109937044135945 -0.025686692856836], PressMdl=[5.48733176777509 -0.092135251339445 -0.0332005633970498 0.773921335537747], Cp=1500, Cv=1200, port_num_NOx=4, NOxMdl=[-0.0710772115732251 13.258266248882 2.53650929146028 -4.98871540780321 18.9690745540948 3.51983329140351 7.35640722696346 -29.5494146545499 -12.7663876549855 -0.0214097840965915 0.143608010417368 -1.21453634962735 0.541720620436424 -0.0774873942784366 -0.515304310267613]}
      mask prompts: Displ "displacement"; CompRatio "compression ratio"; Ncyl "number of cylinders"; ValveMdl "valve model"; TmpMdl "temperature model"; IgnitMdl "ignition model"; PressMdl "pressure model"; port_num_NOx "Model NOx output port number"; NOxMdl "NOx parameters"
      mask help: Combustion development
      mask TabNameString: geometry,geometry,geometry,thermodynamics,thermodynamics,thermodynamics,thermodynamics,thermodynamics,thermodynamics,NOx,NOx
      mask Display:
      | port_label('input', 1, 'Pi');
      | port_label('input', 2, 'Pe');
      | port_label('input', 3, 'Ti');
      | port_label('input', 4, 'O2i');
      | port_label('input', 5, 'Ne');
      | port_label('input', 6, 'iq');
      | port_label('input', 7, 'soi');
      | port_label('input', 8, 'ica');
      | port_label('input', 9, 'eca');
      | port_label('input', 10, 'Prail');
      | port_label('output', 1, 'M');
      | port_label('output', 2, 'Te');
      | port_label('output', 3, 'XO2e');
      | port_label('output', 4, 'NOx');
      | port_label('output', 5, 'lambda');
      | port_label('output', 6, 'phi_ign');
      | port_label('output', 7, 'Pcyl');
      | port_label('output', 8, 'Mf');
  Ground : Ground
  Terminator : Terminator
  Terminator1 : Terminator
  Terminator2 : Terminator
  Meng : Outport
  Tout : Outport  Port=2
  XO2out : Outport  Port=3
  outflow : Outport  Port=4
  Mfuel : Outport  Port=5
  tag scope: Engineengine_CylinderPressure=global, Engineengine_NOxEmissions=global
  wires:
  uPR/1 -> Combustion/10
  uECA/1 -> Combustion/9
  uICA/1 -> Combustion/8
  IQ/1 -> Combustion/6
  Combustion/8 -> Mfuel/1
  Combustion/7 -> [Engineengine_CylinderPressure]
  Combustion/6 -> Terminator2/1
  Combustion/5 -> Terminator1/1
  Combustion/1 -> Meng/1
  inflow/1 -> Terminator/1  "flow"
  Ground/1 -> outflow/1
  OmegaEng/1 -> Combustion/5
  Pin/1 -> Combustion/1
  Pout/1 -> Combustion/2
  Combustion/2 -> Tout/1
  Combustion/3 -> XO2out/1
  XO2in/1 -> Combustion/4
  Combustion/4 -> [Engineengine_NOxEmissions]
  [MixTotalInFlow_MixtureTemperature] -> Combustion/3
  uSOI/1 -> Combustion/7

== system Supported_and_unsupported_combinations/Engine/ExhaustManifold ==
  Meng : Inport
  Tin : Inport  Port=2
  XO2in : Inport  Port=3
  inflow : Inport  Port=4
  Mfuel : Inport  Port=5
  Add4 : Sum
  AdiabaticManifoldXO2 : S-Function  FunctionName=orsb_reservoir_adiabatic_XO2  Parameters=V , R , Cp , pinit , Tinit , XO2init ,  EnableBusSupport=off  mask(reservoir adiabatic XO2 ){V=50, R=288.4, Cp=1135, pinit=247140, Tinit=720.22, XO2init=0.15}
      mask prompts: V "reservoir volume [l]"; R "gas constant [J/K/kg]"; Cp "fixed pressure spec heat [J/kg/K]"; pinit "initial pressure [Pa]"; Tinit "initial temperature [K]"; XO2init "initial oxygen mass fraction [-]"
      mask help: Adiabatic reservoir model with pressure, temperature, and oxygen mass fraction as internal states.
      mask TabNameString: General ,General ,General ,Initialization ,Initialization ,Initialization
      mask Display:
      | port_label('input', 1, 'min ');
      | port_label('input', 2, 'mout ');
      | port_label('input', 3, 'Tin ');
      | port_label('input', 4, 'O2min ');
      | port_label('output', 1, 'pout ');
      | port_label('output', 2, 'Tout ');
      | port_label('output', 3, 'XO2out ');
  Conversion_XO2_lambda : Fcn  Expr=u(1) / 0.231362 * (1 + 14.59) / (14.59 * (1 - u(1) / 0.231362))+1
  Product2 : Product  RndMeth=Zero
  Saturation : Saturate  UpperLimit=0.2313  LowerLimit=0
  Pout : Outport
  outflow : Outport  Port=2
  tag scope: EngineExhaustManifold_OutletLambda=global, EngineExhaustManifold_OutletOxygenFraction=global, EngineExhaustManifold_OutletPressure=global, EngineExhaustManifold_OutletTemperature=global
  wires:
  Saturation/1 -> Conversion_XO2_lambda/1
  Add4/1 -> AdiabaticManifoldXO2/1, Product2/1
  Product2/1 -> AdiabaticManifoldXO2/4
  Meng/1 -> Add4/2
  AdiabaticManifoldXO2/1 -> Pout/1, [EngineExhaustManifold_OutletPressure]
  AdiabaticManifoldXO2/2 -> [EngineExhaustManifold_OutletTemperature]
  Tin/1 -> AdiabaticManifoldXO2/3
  AdiabaticManifoldXO2/3 -> Saturation/1, [EngineExhaustManifold_OutletOxygenFraction]
  XO2in/1 -> Product2/2
  inflow/1 -> outflow/1  "flow"
  Mfuel/1 -> Add4/1
  [FlowSplitterTotalOutFlow_Massflow] -> AdiabaticManifoldXO2/2
  Conversion_XO2_lambda/1 -> [EngineExhaustManifold_OutletLambda]

== system Supported_and_unsupported_combinations/Engine/IntakeManifold ==
  Mout : Inport
  inflow : Inport  Port=2
  IsothermalManifoldXO2 : S-Function  FunctionName=orsb_reservoir_isothermal_XO2  Parameters=V , R , Cp , pinit , XO2init ,  EnableBusSupport=off  mask(reservoir isothermal XO2 ){V=41.2801, R=288.4, Cp=1020, pinit=205590, XO2init=0.22}
      mask prompts: V "reservoir volume [l]"; R "gas constant [J/K/kg]"; Cp "fixed pressure spec heat [J/kg/K]"; pinit "initial pressure [Pa]"; XO2init "initial oxygen mass fraction [-]"
      mask help: Isothermal reservoir model with pressure and oxygen mass fraction as internal states.
      mask TabNameString: General ,General ,General ,Initialization ,Initialization
      mask Display:
      | port_label('input', 1, 'min ');
      | port_label('input', 2, 'mout ');
      | port_label('input', 3, 'Tin ');
      | port_label('input', 4, 'O2min ');
      | port_label('output', 1, 'pout ');
      | port_label('output', 2, 'XO2out ');
  Pim : Outport
  XO2out : Outport  Port=2
  outflow : Outport  Port=3
  tag scope: EngineIntakeManifold_OutletPressure=global
  wires:
  Mout/1 -> IsothermalManifoldXO2/2
  IsothermalManifoldXO2/1 -> Pim/1, [EngineIntakeManifold_OutletPressure]
  IsothermalManifoldXO2/2 -> XO2out/1
  inflow/1 -> outflow/1  "flow"
  [MixTotalInFlow_Massflow] -> IsothermalManifoldXO2/1
  [MixTotalInFlow_OxygenFlow] -> IsothermalManifoldXO2/4
  [MixTotalInFlow_MixtureTemperature] -> IsothermalManifoldXO2/3

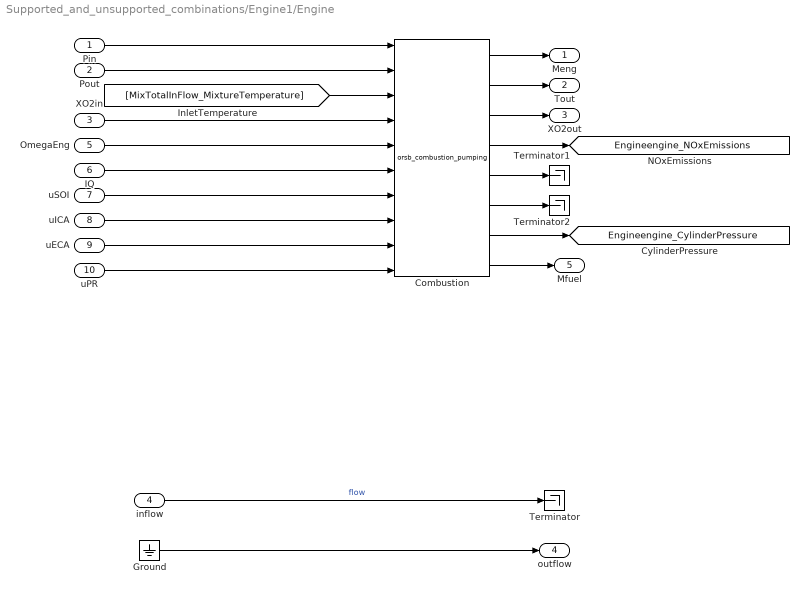
== system Supported_and_unsupported_combinations/Engine1/Engine ==
  Pin : Inport
  Pout : Inport  Port=2
  XO2in : Inport  Port=3
  inflow : Inport  Port=4
  OmegaEng : Inport  Port=5
  IQ : Inport  Port=6
  uSOI : Inport  Port=7
  uICA : Inport  Port=8
  uECA : Inport  Port=9
  uPR : Inport  Port=10
  Combustion : S-Function  FunctionName=orsb_combustion_pumping  Parameters=Displ, CompRatio, Ncyl, ValveMdl, TmpMdl, IgnitMdl, PressMdl, Cp, Cv, port_num_NOx, NOxMdl,  EnableBusSupport=off  mask(combustion_pumping){Displ=12.9, CompRatio=18, Ncyl=6, ValveMdl=[0.00961171539106083 -0.172384589641163], TmpMdl=[-0.025503095647334 0.175522235872159 0.0255043476751577 0.0373865335774022 0], IgnitMdl=[0.484351292851209 0.143524113288744 -0.055676015193126 -0.0109937044135945 -0.025686692856836], PressMdl=[5.48733176777509 -0.092135251339445 -0.0332005633970498 0.773921335537747], Cp=1500, Cv=1200, port_num_NOx=4, NOxMdl=[-0.0710772115732251 13.258266248882 2.53650929146028 -4.98871540780321 18.9690745540948 3.51983329140351 7.35640722696346 -29.5494146545499 -12.7663876549855 -0.0214097840965915 0.143608010417368 -1.21453634962735 0.541720620436424 -0.0774873942784366 -0.515304310267613]}
      mask prompts: Displ "displacement"; CompRatio "compression ratio"; Ncyl "number of cylinders"; ValveMdl "valve model"; TmpMdl "temperature model"; IgnitMdl "ignition model"; PressMdl "pressure model"; port_num_NOx "Model NOx output port number"; NOxMdl "NOx parameters"
      mask help: Combustion development
      mask TabNameString: geometry,geometry,geometry,thermodynamics,thermodynamics,thermodynamics,thermodynamics,thermodynamics,thermodynamics,NOx,NOx
      mask Display:
      | port_label('input', 1, 'Pi');
      | port_label('input', 2, 'Pe');
      | port_label('input', 3, 'Ti');
      | port_label('input', 4, 'O2i');
      | port_label('input', 5, 'Ne');
      | port_label('input', 6, 'iq');
      | port_label('input', 7, 'soi');
      | port_label('input', 8, 'ica');
      | port_label('input', 9, 'eca');
      | port_label('input', 10, 'Prail');
      | port_label('output', 1, 'M');
      | port_label('output', 2, 'Te');
      | port_label('output', 3, 'XO2e');
      | port_label('output', 4, 'NOx');
      | port_label('output', 5, 'lambda');
      | port_label('output', 6, 'phi_ign');
      | port_label('output', 7, 'Pcyl');
      | port_label('output', 8, 'Mf');
  Ground : Ground
  Terminator : Terminator
  Terminator1 : Terminator
  Terminator2 : Terminator
  Meng : Outport
  Tout : Outport  Port=2
  XO2out : Outport  Port=3
  outflow : Outport  Port=4
  Mfuel : Outport  Port=5
  tag scope: Engineengine_CylinderPressure=global, Engineengine_NOxEmissions=global
  wires:
  uSOI/1 -> Combustion/7
  [MixTotalInFlow_MixtureTemperature] -> Combustion/3
  Combustion/4 -> [Engineengine_NOxEmissions]
  XO2in/1 -> Combustion/4
  Combustion/3 -> XO2out/1
  Combustion/2 -> Tout/1
  Pout/1 -> Combustion/2
  Pin/1 -> Combustion/1
  OmegaEng/1 -> Combustion/5
  Ground/1 -> outflow/1
  inflow/1 -> Terminator/1  "flow"
  Combustion/1 -> Meng/1
  Combustion/5 -> Terminator1/1
  Combustion/6 -> Terminator2/1
  Combustion/7 -> [Engineengine_CylinderPressure]
  Combustion/8 -> Mfuel/1
  IQ/1 -> Combustion/6
  uICA/1 -> Combustion/8
  uECA/1 -> Combustion/9
  uPR/1 -> Combustion/10

== system Supported_and_unsupported_combinations/Engine1/ExhaustManifold ==
  Meng : Inport
  Tin : Inport  Port=2
  XO2in : Inport  Port=3
  inflow : Inport  Port=4
  Mfuel : Inport  Port=5
  Add4 : Sum
  AdiabaticManifoldXO2 : S-Function  FunctionName=orsb_reservoir_adiabatic_XO2  Parameters=V , R , Cp , pinit , Tinit , XO2init ,  EnableBusSupport=off  mask(reservoir adiabatic XO2 ){V=50, R=288.4, Cp=1135, pinit=247140, Tinit=720.22, XO2init=0.15}
      mask prompts: V "reservoir volume [l]"; R "gas constant [J/K/kg]"; Cp "fixed pressure spec heat [J/kg/K]"; pinit "initial pressure [Pa]"; Tinit "initial temperature [K]"; XO2init "initial oxygen mass fraction [-]"
      mask help: Adiabatic reservoir model with pressure, temperature, and oxygen mass fraction as internal states.
      mask TabNameString: General ,General ,General ,Initialization ,Initialization ,Initialization
      mask Display:
      | port_label('input', 1, 'min ');
      | port_label('input', 2, 'mout ');
      | port_label('input', 3, 'Tin ');
      | port_label('input', 4, 'O2min ');
      | port_label('output', 1, 'pout ');
      | port_label('output', 2, 'Tout ');
      | port_label('output', 3, 'XO2out ');
  Conversion_XO2_lambda : Fcn  Expr=u(1) / 0.231362 * (1 + 14.59) / (14.59 * (1 - u(1) / 0.231362))+1
  Product2 : Product  RndMeth=Zero
  Saturation : Saturate  UpperLimit=0.2313  LowerLimit=0
  Pout : Outport
  outflow : Outport  Port=2
  tag scope: EngineExhaustManifold_OutletLambda=global, EngineExhaustManifold_OutletOxygenFraction=global, EngineExhaustManifold_OutletPressure=global, EngineExhaustManifold_OutletTemperature=global
  wires:
  Conversion_XO2_lambda/1 -> [EngineExhaustManifold_OutletLambda]
  [FlowSplitterTotalOutFlow_Massflow] -> AdiabaticManifoldXO2/2
  Mfuel/1 -> Add4/1
  inflow/1 -> outflow/1  "flow"
  XO2in/1 -> Product2/2
  AdiabaticManifoldXO2/3 -> [EngineExhaustManifold_OutletOxygenFraction], Saturation/1
  Tin/1 -> AdiabaticManifoldXO2/3
  AdiabaticManifoldXO2/2 -> [EngineExhaustManifold_OutletTemperature]
  AdiabaticManifoldXO2/1 -> [EngineExhaustManifold_OutletPressure], Pout/1
  Meng/1 -> Add4/2
  Product2/1 -> AdiabaticManifoldXO2/4
  Add4/1 -> Product2/1, AdiabaticManifoldXO2/1
  Saturation/1 -> Conversion_XO2_lambda/1

== system Supported_and_unsupported_combinations/Engine1/IntakeManifold ==
  Mout : Inport
  inflow : Inport  Port=2
  IsothermalManifoldXO2 : S-Function  FunctionName=orsb_reservoir_isothermal_XO2  Parameters=V , R , Cp , pinit , XO2init ,  EnableBusSupport=off  mask(reservoir isothermal XO2 ){V=41.2801, R=288.4, Cp=1020, pinit=205590, XO2init=0.22}
      mask prompts: V "reservoir volume [l]"; R "gas constant [J/K/kg]"; Cp "fixed pressure spec heat [J/kg/K]"; pinit "initial pressure [Pa]"; XO2init "initial oxygen mass fraction [-]"
      mask help: Isothermal reservoir model with pressure and oxygen mass fraction as internal states.
      mask TabNameString: General ,General ,General ,Initialization ,Initialization
      mask Display:
      | port_label('input', 1, 'min ');
      | port_label('input', 2, 'mout ');
      | port_label('input', 3, 'Tin ');
      | port_label('input', 4, 'O2min ');
      | port_label('output', 1, 'pout ');
      | port_label('output', 2, 'XO2out ');
  Pim : Outport
  XO2out : Outport  Port=2
  outflow : Outport  Port=3
  tag scope: EngineIntakeManifold_OutletPressure=global
  wires:
  [MixTotalInFlow_MixtureTemperature] -> IsothermalManifoldXO2/3
  [MixTotalInFlow_OxygenFlow] -> IsothermalManifoldXO2/4
  [MixTotalInFlow_Massflow] -> IsothermalManifoldXO2/1
  inflow/1 -> outflow/1  "flow"
  IsothermalManifoldXO2/2 -> XO2out/1
  IsothermalManifoldXO2/1 -> [EngineIntakeManifold_OutletPressure], Pim/1
  Mout/1 -> IsothermalManifoldXO2/2
